simulink model "EGH446"  (R2020a)
settings: Solver=ode45  StartTime=0.0  StopTime=inf  RelTol=1e-5  EnableMultiTasking=on
PreLoadFcn:
  | ModelStartup
InitFcn:
  | load('sim_parameters')
  | load('complexMap.mat')
StartFcn:
  | drawPath
StopFcn:
  | drawPath
values from neighbouring files (symbols this model uses):
  dt = distanceTransform(x,[46,20])    [MapTest.m]
  obstacles = [4 8 8 8 2 14 22 16 23 24 12 21 ... (36 elements, 12x3)]    [obstacles.mat]
  path = [nodeRow(currentNode) nodeCol(currentNode); path]    [Astar.m]    (also in ModelStartup.m = [path(1:i-2,:); path(i:end,:)]; PathPlanning.m = [path; current])
  wpList = getWaypoints(NWaypoints,inflatedMap, obstacles, xmax,ymax)    [ModelStartup.m]
undefined symbols (not defined in the file or in its folder): DiscIntNeverNeededParam, Ke, mot_B, mot_COM, pp_cont, Ts, veh
libraries: mobileRoboticsLib x3, simulink_extras x3, simulink x3
PauseFcn:
  | drawPath
settings Model: SimulationMode=accelerator  Creator=sriramn  LastModifiedBy=CodyS
settings SolverCC: ZeroCrossAlgorithm=Adaptive
settings DataIOCC: LimitDataPoints=on  SaveFormat=Array  ReturnWorkspaceOutputs=off
settings OptimizationCC: LifeSpan=inf
settings DebuggingCC: SolverPrmCheckMsg=warning  AllowSymbolicDim=off  SFUnexpectedBacktrackingDiag=warning  SFNoUnconditionalDefaultTransitionDiag=warning  SFExecutionAtInitializationDiag=none  ArithmeticOperatorsInVariantConditions=warning
settings HardwareCC: ProdBitPerPointer=32  ProdBitPerSizeT=32  ProdBitPerPtrDiffT=32  ProdLargestAtomicFloat=None  ProdIntDivRoundTo=Undefined  ProdEndianess=Unspecified  ProdWordSize=32  ProdHWDeviceType=32-bit Generic
settings ModelReferenceCC: ModelReferenceMinAlgLoopOccurrences=on  PropagateSignalLabelsOutOfModel=off
settings SFSimCC: SimUseLocalCustomCode=off  CustomCodeUndefinedFunction=UseInterfaceOnly
settings RTWCC: RTWUseLocalCustomCode=off
settings CodeAppCC: StateflowObjectComments=on
settings GRTTargetCC: TargetLangStandard=C89/C90 (ANSI)
settings ConfigComp: CovMetricSettings=dw  CovHtmlReporting=on  CovSaveCumulativeToWorkspaceVar=on  CovSaveSingleToWorkspaceVar=on  CovExternalEMLEnable=off  CovSFcnEnable=off
settings SimscapeCC: SimscapeNormalizeSystem=off
settings ConfigurationSet: Description=SimMechanics 2G
settings ExplorerConfigSet: InternalSimMechanicsExplorerSettings="<ExplorerConfiguration><canonicalview>planar_xy</canonicalview><AnimationSetting><BasePlaybackSpeed>1.0</BasePlaybackSpeed><PlaybackSpeedFactor>1.0</PlaybackSpeedFactor></AnimationSetting><TilePanel><TileInfo><Tiles Columns=\"1\" Count=\"1\" Rows=\"1\"><Column Left=\"2\" Weight=\"1\"/><Column Left=\"1628\"/><Row Top=\"2\" Weight=\"1\"/><Row Top=\"1072\"/><Tile Height=\"1\" Width=\"1\" X=\"0\" Y=\"0\"/></Tiles></TileInfo><SceneInfo><SceneViewer><BGColor><R>0.60000002384185791</R><G>0.60000002384185791</G><B>0.60000002384185791</B></BGColor><Camera><Position><X>0.22951840878551699</X><Y>0.32651610611526627</Y><Z>-0.27215421354393321</Z></Position><Center><X>-0.15775714411666431</X><Y>-0.15462825985839526</Y><Z>0.065702552916005602</Z></Center><Up><X>-0.56030137557930915</X><Y>0.72817587161684794</Y><Z>0.39474329445726858</Z></Up><Left>-0.21481383955700509</Left><Right>0.21481383955700509</Right><Bottom>-0.27569784609469139</Bottom><Top>0.27569784609469139</Top></Camera></SceneViewer></SceneInfo></TilePanel></ExplorerConfiguration>"

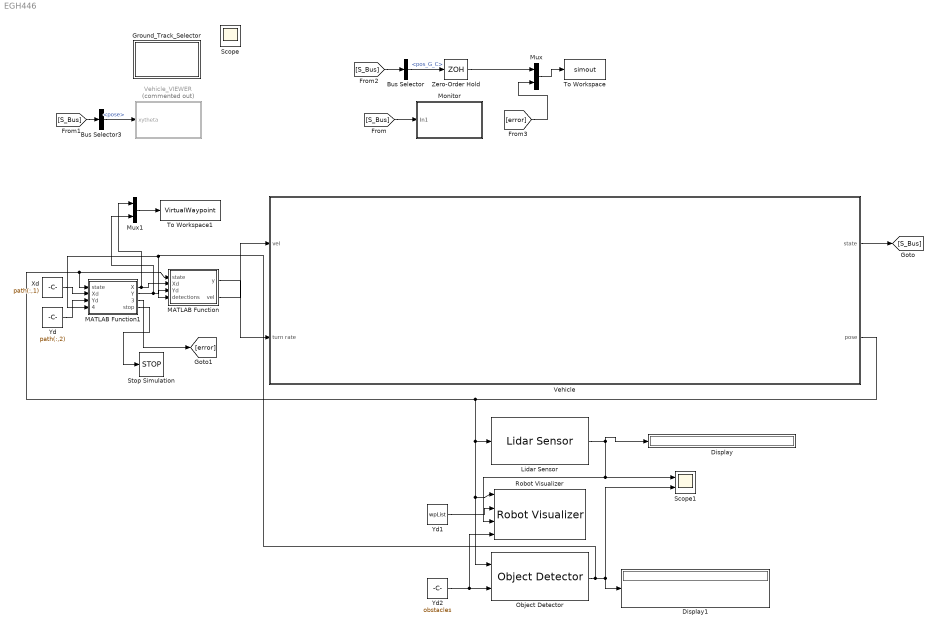
== system EGH446 ==
  Bus Selector : BusSelector  OutputSignals=BUS_G_frame.pos_G_C
  Bus Selector3 : BusSelector  OutputSignals=pose
  Display : Display
  Display1 : Display
  Ground_Track_Selector : Subsystem  mask{the_XL_filename=ground_robot_waypoints.xlsx, the_racetrack_str=SMALL_S_HOME, the_look_ahead_dist=0.260, the_des_lin_vel=0.1, the_max_ang_vel_deg_sec=60}
      mask prompts: the_XL_filename "EXCEL file (eg: bh.xlsx)"; the_racetrack_str "Racetrack type"; the_look_ahead_dist "Look ahead distance (m)"; the_des_lin_vel "Desired Linear Velocity (m/sec)"; the_max_ang_vel_deg_sec "Max Angular Velocity (deg/sec)"
      mask init:
      | %fprintf('\n ... <%s> and <%s>',the_XL_filename, the_racetrack_str);
      | 
      | A_MASK_OBJ  = Simulink.Mask.get(gcb);
      | A_IMAGE_OBJ = A_MASK_OBJ.getDialogControl('the_track_pic_param');
      | A_IMAGE_OBJ.FilePath = [the_racetrack_str,'.png'];
      | 
      | %--------------------------------------------------------------
      | THE_FILE  = the_XL_filename; 
      | THE_SHEET = the_racetrack_str;
      | my_path_data_T = readtable(THE_FILE, 'Sheet', THE_SHEET);
      | 
      | assignin('base', 'my_path_data_T', my_path_data_T );
      | evalin(  'base', 'pp_cont.Waypoints = [my_path_data_T.X,  my_path_data_T.Y ];' );
      | evalin('base', 'close all');
      | %--------------------------------------------------------------
      | evalin('base', ['pp_cont.LookaheadDistance=',num2str(the_look_ahead_dist),';']);
      | evalin('base', ['pp_cont.DesiredLinearVelocity=',num2str(the_des_lin_vel),';']);
      | evalin('base', ['pp_cont.MaxAngularVelocity=',num2str(the_max_ang_vel_deg_sec*pi/180),';']);
      | %pp_cont.LookaheadDistance     = 0.2;        % m 
      | %pp_cont.DesiredLinearVelocity = 0.1;        % m/s
      | %pp_cont.MaxAngularVelocity    = 60*pi/180;  %radians/second
      mask TypeOptions the_racetrack_str: SPANNER | RECT_TRI | MEDIUM_S_HOME | SMALL_S_HOME | SQUARE | CIRCLE_HOME | L_AND_R_TURNS | Assignment PartA | Tuning
      mask DialogControl DescGroupVar Prompt: m_RaceTrack_Selector
      mask DialogControl DescTextVar Prompt: Select the racetrack for your Differential Drive Robot (DDR).  And specify the parameters for your Pure Pursuit controller.
      mask DialogControl Container10 Prompt: RaceTrack
      mask DialogControl Container5 Prompt: PurePursuit
      mask DialogControl Control4 Prompt: If you want some DEFAULT values then click on the button below
      mask DialogControl the_set_def_PP_values Prompt: Set Default values
      mask DialogControl the_set_def_PP_values Callback:
      | set_param(gcb,'the_look_ahead_dist','0.2');
      | set_param(gcb,'the_des_lin_vel','0.1');
      | set_param(gcb,'the_max_ang_vel_deg_sec','60');
      | fprintf('\n *** applied DEFAULT values to PP params ***');
      mask DialogControl Control2 Prompt: As a general rule, the lookahead distance should be larger than the desired linear velocity for a smooth path. The robot might cut corners when the lookahead distance is large. In contrast, a small lookahead distance can result in an unstable path following behavior.
      mask Display: fprintf('%s',the_racetrack_str)
  Lidar Sensor : mobileRoboticsLib/Environments/Lidar Sensor  mapName=map  sensorOffset=[ 0, 0 ]  scanAngles=[ -pi/4, 0, pi/4 ]  maxRange=5
      settings: SourceProductName=Mobile Robotics Simulation Toolbox
  MATLAB Function : MATLAB Function  TreatAsAtomicUnit=on
  MATLAB Function1 : MATLAB Function  TreatAsAtomicUnit=on
  Monitor : Subsystem
  Mux : Mux  Inputs=2
  Mux1 : Mux  Inputs=2
  Object Detector : mobileRoboticsLib/Environments/Object Detector  sensorOffset=[ 0, 0 ]  sensorAngle=0  fieldOfView=pi/3  maxRange=5  maxDetections=3  sampleTime=0.1
      settings: SourceProductName=Mobile Robotics Simulation Toolbox
  Robot Visualizer : mobileRoboticsLib/Environments/Robot Visualizer  robotRadius=0  mapName=map  showTrajectory=on  hasWaypoints=on  hasLidar=on  sensorOffset=[ 0, 0 ]  scanAngles=[ -pi/4, 0, pi/4 ]  hasObjDetector=on  objDetectorOffset=[ 0, 0 ]  objDetectorAngle=0  objDetectorFOV=pi/4  objDetectorMaxRange=5  objectColors=[ 1, 0, 0; 0, 1, 0; 0, 0, 1 ]  objectMarkers=s
  Scope1 : Scope  NumInputPorts=2
  Stop Simulation : Stop
  To Workspace : ToWorkspace  VariableName=simout  SaveFormat=Structure With Time  SampleTime=-1
  To Workspace1 : ToWorkspace  VariableName=VirtualWaypoint  SampleTime=-1
  Vehicle : Subsystem
  Vehicle_VIEWER : Subsystem  Commented=on  mask{wp_mat=pp_cont.Waypoints, veh_ID_num=1, veh_init_xytheta=veh.states.init_pose, Ts=0.1}
      mask prompts: wp_mat "Waypoint matrix for arena [x_col, y_col] (m)"; veh_ID_num "Vehicle ID number"; veh_init_xytheta "Initial pose [x,y,theta]"; Ts "Sample time for updating animation (secs)"
      mask TypeOptions veh_ID_num: 1 | 2 | 3 | 4
      mask DialogControl Control2 Prompt: Animate simulation of Differential Drive Robot (DDR)
      mask Display: fprintf('veh_ID=%d',veh_ID_num);
  Xd : Constant  Value=path(:,1)
  Yd : Constant  Value=path(:,2)
  Yd1 : Constant  Value=wpList
  Yd2 : Constant  Value=obstacles
  Zero-Order Hold : ZeroOrderHold  SampleTime=0.01
  Scope : Scope
  wires:
  [S_Bus] -> Bus Selector3/1
  Bus Selector/1 -> Zero-Order Hold/1  "<pos_G_C>"
  Zero-Order Hold/1 -> Mux/1
  [S_Bus] -> Monitor/1(In1)
  Bus Selector3/1 -> Vehicle_VIEWER/1(xytheta)  "<pose>"
  [S_Bus] -> Bus Selector/1
  Vehicle/1(state) -> [S_Bus]
  MATLAB Function/1(y) -> Vehicle/2(turn rate)
  Vehicle/2(pose) -> Object Detector/1, Robot Visualizer/1, Lidar Sensor/1, MATLAB Function1/1(state), MATLAB Function/1(state)
  MATLAB Function/2(vel) -> Vehicle/1(vel)
  Xd/1 -> MATLAB Function1/2(Xd)
  Yd/1 -> MATLAB Function1/3(Yd)
  MATLAB Function1/1(X) -> Mux1/1, MATLAB Function/2(Xd)
  MATLAB Function1/2(Y) -> Mux1/2, MATLAB Function/3(Yd)
  MATLAB Function1/3(d_error) -> [error]
  MATLAB Function1/4(stop) -> Stop Simulation/1
  [error] -> Mux/2
  Mux/1 -> To Workspace/1
  Yd1/1 -> Robot Visualizer/2
  Yd2/1 -> Robot Visualizer/4, Object Detector/2
  Object Detector/1 -> MATLAB Function1/4(detections), MATLAB Function/4(detections), Scope1/2, Display1/1
  Lidar Sensor/1 -> Scope1/1, Robot Visualizer/3, Display/1
  Mux1/1 -> To Workspace1/1

== system EGH446/Ground_Track_Selector ==

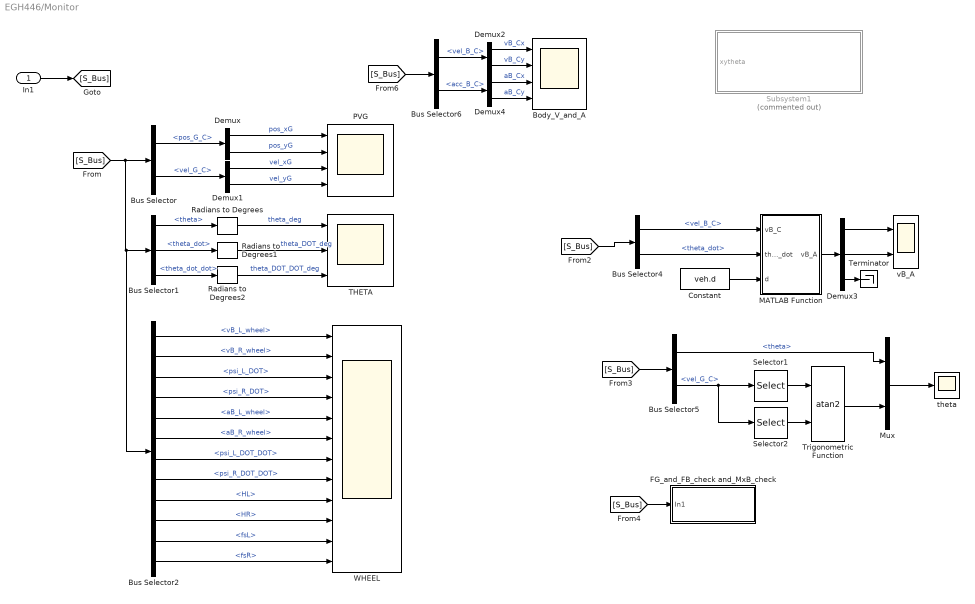
== system EGH446/Monitor ==
  In1 : Inport
  Body_V_and_A : Scope  NumInputPorts=4
  Bus Selector : BusSelector  OutputSignals=BUS_G_frame.pos_G_C,BUS_G_frame.vel_G_C
  Bus Selector1 : BusSelector  OutputSignals=theta,theta_dot,theta_dot_dot
  Bus Selector2 : BusSelector  OutputSignals=BUS_wheel.BUS_wheel_vel.vB_L_wheel,BUS_wheel.BUS_wheel_vel.vB_R_wheel,BUS_wheel.BUS_wheel_vel.psi_L_DOT,BUS_wheel.BUS_wheel_vel.psi_R_DOT,BUS_wheel.BUS_wheel_acc.aB_L_wheel,BUS_wheel.BUS_wheel_acc.aB_R_wheel,BUS_wheel.BUS_wheel_acc.psi_L_DOT_DOT,BUS_wheel.BUS_wheel_acc.psi_R_DOT_DOT,BUS_wheel.BUS_wheel_force.HL,BUS_wheel.BUS_wheel_force.HR,BUS_wheel.BUS_wheel_force.fsL,BUS_wheel.BUS_wheel_force.fsR
  Bus Selector4 : BusSelector  OutputSignals=BUS_B_frame.vel_B_C,theta_dot
  Bus Selector5 : BusSelector  OutputSignals=theta,BUS_G_frame.vel_G_C
  Bus Selector6 : BusSelector  OutputSignals=BUS_B_frame.vel_B_C,BUS_B_frame.acc_B_C
  Constant : Constant  Value=veh.d
  Demux{,1..2,4} (4 alike) : Demux  Outputs=2
  Demux3 : Demux  Outputs=3
  FG_and_FB_check and_MxB_check : Subsystem
  MATLAB Function : MATLAB Function  TreatAsAtomicUnit=on
  Mux : Mux  Inputs=2
  PVG : Scope  NumInputPorts=4
  Radians to Degrees : simulink_extras/Transformations/Radians to Degrees
  Radians to Degrees1 : simulink_extras/Transformations/Radians to Degrees
  Radians to Degrees2 : simulink_extras/Transformations/Radians to Degrees
  Selector1 : Selector  InputPortWidth=2  IndexOptions=Index vector (dialog)  Indices=[ 2]  OutputSizes=1
  Selector2 : Selector  InputPortWidth=2  IndexOptions=Index vector (dialog)  Indices=[ 1]  OutputSizes=1
  Subsystem1 : Subsystem  Commented=on  mask{wp_mat=[0, 1, 1, 0, 0, 1; 0,0,0.5,0.5,1,1]', veh_ID_num=2, veh_init_xytheta=[0,0,0], Ts=0.1}
      mask prompts: wp_mat "Waypoint matrix for arena [x_col, y_col] (m)"; veh_ID_num "Vehicle ID number"; veh_init_xytheta "Initial pose [x,y,theta]"; Ts "Sample time for updating animation (secs)"
      mask TypeOptions veh_ID_num: 1 | 2 | 3 | 4
      mask DialogControl Control2 Prompt: Animate simulation of Differential Drive Robot (DDR)
      mask Display: fprintf('veh_ID=%d',veh_ID_num);
  THETA : Scope  NumInputPorts=3
  Terminator : Terminator
  Trigonometric Function : Trigonometry  Operator=atan2
  WHEEL : Scope  NumInputPorts=12
  theta : Scope
  vB_A : Scope  NumInputPorts=2
  wires:
  In1/1 -> [S_Bus]
  [S_Bus] -> Bus Selector2/1, Bus Selector1/1, Bus Selector/1
  Bus Selector/1 -> Demux/1  "<pos_G_C>"
  Demux/1 -> PVG/1  "pos_xG"
  Demux/2 -> PVG/2  "pos_yG"
  Bus Selector/2 -> Demux1/1  "<vel_G_C>"
  Demux1/1 -> PVG/3  "vel_xG"
  Demux1/2 -> PVG/4  "vel_yG"
  Bus Selector1/1 -> Radians to Degrees/1  "<theta>"
  Radians to Degrees2/1 -> THETA/3  "theta_DOT_DOT_deg"
  Radians to Degrees1/1 -> THETA/2  "theta_DOT_deg"
  Radians to Degrees/1 -> THETA/1  "theta_deg"
  Bus Selector1/2 -> Radians to Degrees1/1  "<theta_dot>"
  Bus Selector1/3 -> Radians to Degrees2/1  "<theta_dot_dot>"
  Bus Selector2/5 -> WHEEL/5  "<aB_L_wheel>"
  Bus Selector2/9 -> WHEEL/9  "<HL>"
  Bus Selector2/7 -> WHEEL/7  "<psi_L_DOT_DOT>"
  Bus Selector2/2 -> WHEEL/2  "<vB_R_wheel>"
  Bus Selector2/4 -> WHEEL/4  "<psi_R_DOT>"
  Bus Selector2/6 -> WHEEL/6  "<aB_R_wheel>"
  Bus Selector2/8 -> WHEEL/8  "<psi_R_DOT_DOT>"
  Bus Selector2/3 -> WHEEL/3  "<psi_L_DOT>"
  Bus Selector2/1 -> WHEEL/1  "<vB_L_wheel>"
  Bus Selector2/10 -> WHEEL/10  "<HR>"
  Bus Selector2/11 -> WHEEL/11  "<fsL>"
  Bus Selector2/12 -> WHEEL/12  "<fsR>"
  [S_Bus] -> Bus Selector4/1
  Bus Selector4/1 -> MATLAB Function/1(vB_C)  "<vel_B_C>"
  [S_Bus] -> Bus Selector5/1
  Bus Selector5/2 -> Selector1/1, Selector2/1  "<vel_G_C>"
  Selector2/1 -> Trigonometric Function/2
  Selector1/1 -> Trigonometric Function/1
  Trigonometric Function/1 -> Mux/2
  Bus Selector5/1 -> Mux/1  "<theta>"
  Mux/1 -> theta/1
  Bus Selector4/2 -> MATLAB Function/2(theta_dot)  "<theta_dot>"
  Constant/1 -> MATLAB Function/3(d)
  MATLAB Function/1(vB_A) -> Demux3/1
  Demux3/3 -> Terminator/1
  Demux3/1 -> vB_A/1
  Demux3/2 -> vB_A/2
  [S_Bus] -> Bus Selector6/1
  Demux4/1 -> Body_V_and_A/3  "aB_Cx"
  Demux4/2 -> Body_V_and_A/4  "aB_Cy"
  Bus Selector6/1 -> Demux2/1  "<vel_B_C>"
  Bus Selector6/2 -> Demux4/1  "<acc_B_C>"
  Demux2/2 -> Body_V_and_A/2  "vB_Cy"
  Demux2/1 -> Body_V_and_A/1  "vB_Cx"
  [S_Bus] -> FG_and_FB_check and_MxB_check/1(In1)

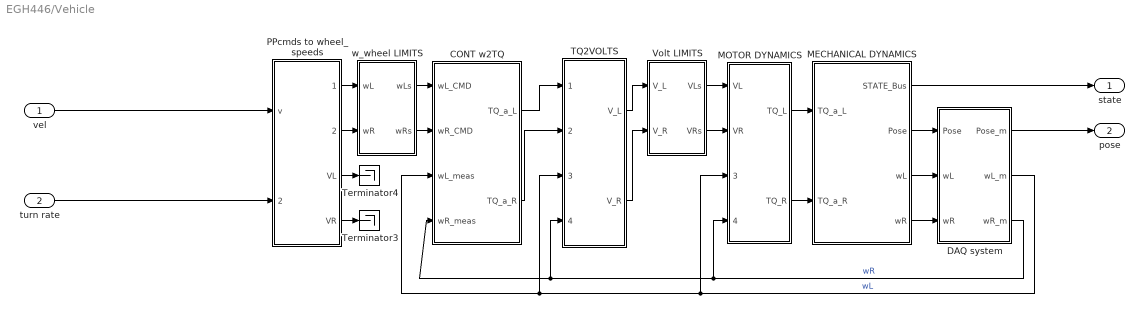
== system EGH446/Vehicle ==
  vel : Inport
  turn rate : Inport  Port=2
  CONT w2TQ : Subsystem
  DAQ system : Subsystem
  MECHANICAL DYNAMICS : Subsystem
      mask Display: image(imread('bh_pics_veh_01.JPG'));
  MOTOR DYNAMICS : Subsystem
  PPcmds to wheel_speeds : Subsystem  mask(PP_cmds_to_Wheel_vels){r=veh.wheel.r, L=veh.L_half_axle}
      mask prompts: r "Radius (r) of driving wheels (m)"; L "Axle HALF length (L) separating wheels  (m)"
      mask help: Convert Pure Pursuit commands into WHEEL velocities.
      mask DialogControl Container10 Prompt: GEOMETRY
  TQ2VOLTS : Subsystem
  Terminator3 : Terminator
  Terminator4 : Terminator
  Volt LIMITS : Subsystem
      mask Display: image(imread('bh_sat.JPG'), [0.25 0.25 0.5 0.5])
  w_wheel LIMITS : Subsystem
      mask Display: image(imread('bh_sat.JPG'), [0.25 0.25 0.5 0.5])
  state : Outport  VectorParamsAs1DForOutWhenUnconnected=off
  pose : Outport  Port=2  VectorParamsAs1DForOutWhenUnconnected=off
  wires:
  turn rate/1 -> PPcmds to wheel_speeds/2(theta_DOT)
  vel/1 -> PPcmds to wheel_speeds/1(v)
  PPcmds to wheel_speeds/4(VR) -> Terminator3/1
  CONT w2TQ/1(TQ_a_L) -> TQ2VOLTS/1(TL_cmd)
  TQ2VOLTS/2(V_R) -> Volt LIMITS/2(V_R)
  DAQ system/1(Pose_m) -> pose/1
  MOTOR DYNAMICS/2(TQ_R) -> MECHANICAL DYNAMICS/2(TQ_a_R)
  Volt LIMITS/1(VLs) -> MOTOR DYNAMICS/1(VL)
  PPcmds to wheel_speeds/3(VL) -> Terminator4/1
  PPcmds to wheel_speeds/1(wL_wheel) -> w_wheel LIMITS/1(wL)
  TQ2VOLTS/1(V_L) -> Volt LIMITS/1(V_L)
  MECHANICAL DYNAMICS/1(STATE_Bus) -> state/1
  Volt LIMITS/2(VRs) -> MOTOR DYNAMICS/2(VR)
  w_wheel LIMITS/2(wRs) -> CONT w2TQ/2(wR_CMD)
  w_wheel LIMITS/1(wLs) -> CONT w2TQ/1(wL_CMD)
  DAQ system/3(wR_m) -> CONT w2TQ/4(wR_meas), TQ2VOLTS/4(wR_meas), MOTOR DYNAMICS/4(wR_meas)  "wR"
  CONT w2TQ/2(TQ_a_R) -> TQ2VOLTS/2(TR_cmd)
  MECHANICAL DYNAMICS/3(wL) -> DAQ system/2(wL)
  MOTOR DYNAMICS/1(TQ_L) -> MECHANICAL DYNAMICS/1(TQ_a_L)
  MECHANICAL DYNAMICS/2(Pose) -> DAQ system/1(Pose)
  DAQ system/2(wL_m) -> CONT w2TQ/3(wL_meas), TQ2VOLTS/3(wL_meas), MOTOR DYNAMICS/3(wL_meas)  "wL"
  PPcmds to wheel_speeds/2(wR_wheel) -> w_wheel LIMITS/2(wR)
  MECHANICAL DYNAMICS/4(wR) -> DAQ system/3(wR)

== system EGH446/Vehicle_VIEWER ==
  xytheta : Inport
  Level-2 MATLAB S-Function : M-S-Function  FunctionName=bh_ddr_animate_sfun  Parameters=Ts, wp_mat, veh_ID_num, veh_init_xytheta
  Signal Specification : SignalSpecification  Dimensions=3
  wires:
  xytheta/1 -> Signal Specification/1
  Signal Specification/1 -> Level-2 MATLAB S-Function/1

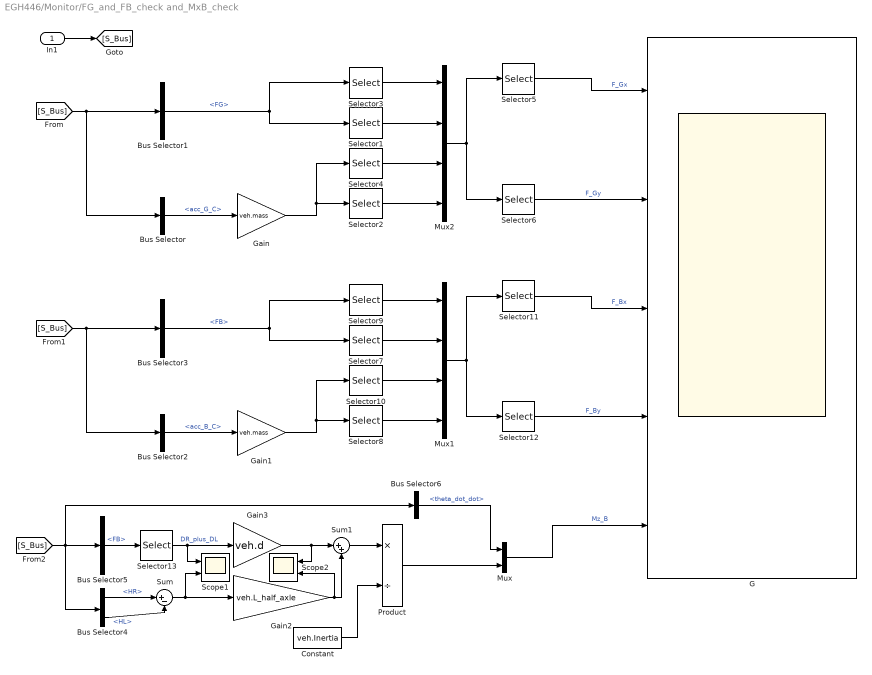
== system EGH446/Monitor/FG_and_FB_check and_MxB_check ==
  In1 : Inport
  Bus Selector : BusSelector  OutputSignals=BUS_G_frame.acc_G_C
  Bus Selector1 : BusSelector  OutputSignals=BUS_veh_F.BUS_veh_FG.FG
  Bus Selector2 : BusSelector  OutputSignals=BUS_B_frame.acc_B_C
  Bus Selector3 : BusSelector  OutputSignals=BUS_veh_F.BUS_veh_Fb.FB
  Bus Selector4 : BusSelector  OutputSignals=BUS_wheel.BUS_wheel_force.HR,BUS_wheel.BUS_wheel_force.HL
  Bus Selector5 : BusSelector  OutputSignals=BUS_veh_F.BUS_veh_Fb.FB
  Bus Selector6 : BusSelector  OutputSignals=theta_dot_dot
  Constant : Constant  Value=veh.Inertia
  G : Scope  NumInputPorts=5
  Gain : Gain  Gain=veh.mass
  Gain1 : Gain  Gain=veh.mass
  Gain2 : Gain  Gain=veh.L_half_axle
  Gain3 : Gain  Gain=veh.d
  Mux : Mux  Inputs=2
  Mux1 : Mux
  Mux2 : Mux
  Product : Product  Inputs=*/
  Scope1 : Scope  NumInputPorts=2
  Scope2 : Scope  NumInputPorts=2
  Selector{1..2,7..8,13} (5 alike) : Selector  InputPortWidth=2  IndexOptions=Index vector (dialog)  Indices=2  OutputSizes=1
  Selector{3..4,9..10} (4 alike) : Selector  InputPortWidth=2  IndexOptions=Index vector (dialog)  Indices=1  OutputSizes=1
  Selector11 : Selector  InputPortWidth=4  IndexOptions=Index vector (dialog)  Indices=[1 3]  OutputSizes=1
  Selector12 : Selector  InputPortWidth=4  IndexOptions=Index vector (dialog)  Indices=[2 4]  OutputSizes=1
  Selector5 : Selector  InputPortWidth=4  IndexOptions=Index vector (dialog)  Indices=[1 3]  OutputSizes=1
  Selector6 : Selector  InputPortWidth=4  IndexOptions=Index vector (dialog)  Indices=[2 4]  OutputSizes=1
  Sum : Sum  Inputs=|+-
  Sum1 : Sum  Inputs=|++
  wires:
  In1/1 -> [S_Bus]
  [S_Bus] -> Bus Selector/1, Bus Selector1/1
  Bus Selector/1 -> Gain/1  "<acc_G_C>"
  Gain/1 -> Selector4/1, Selector2/1
  Selector3/1 -> Mux2/1
  Selector1/1 -> Mux2/2
  Selector4/1 -> Mux2/3
  Selector2/1 -> Mux2/4
  Mux2/1 -> Selector5/1, Selector6/1
  Selector6/1 -> G/2  "F_Gy"
  Selector5/1 -> G/1  "F_Gx"
  Bus Selector1/1 -> Selector3/1, Selector1/1  "<FG>"
  [S_Bus] -> Bus Selector2/1, Bus Selector3/1
  Bus Selector2/1 -> Gain1/1  "<acc_B_C>"
  Gain1/1 -> Selector10/1, Selector8/1
  Selector9/1 -> Mux1/1
  Selector7/1 -> Mux1/2
  Selector10/1 -> Mux1/3
  Selector8/1 -> Mux1/4
  Mux1/1 -> Selector11/1, Selector12/1
  Selector12/1 -> G/4  "F_By"
  Selector11/1 -> G/3  "F_Bx"
  Bus Selector3/1 -> Selector9/1, Selector7/1  "<FB>"
  [S_Bus] -> Bus Selector6/1, Bus Selector4/1, Bus Selector5/1
  Bus Selector5/1 -> Selector13/1  "<FB>"
  Selector13/1 -> Scope1/1, Gain3/1  "DR_plus_DL"
  Sum/1 -> Scope1/2, Gain2/1
  Gain3/1 -> Scope2/1, Sum1/1
  Gain2/1 -> Scope2/2, Sum1/2
  Mux/1 -> G/5  "Mz_B"
  Product/1 -> Mux/2
  Constant/1 -> Product/2
  Sum1/1 -> Product/1
  Bus Selector4/1 -> Sum/1  "<HR>"
  Bus Selector4/2 -> Sum/2  "<HL>"
  Bus Selector6/1 -> Mux/1  "<theta_dot_dot>"

== system EGH446/Monitor/Subsystem1 ==
  xytheta : Inport
  Level-2 MATLAB S-Function : M-S-Function  FunctionName=bh_ddr_animate_sfun  Parameters=Ts, wp_mat, veh_ID_num, veh_init_xytheta
  Signal Specification : SignalSpecification  Dimensions=3
  wires:
  xytheta/1 -> Signal Specification/1
  Signal Specification/1 -> Level-2 MATLAB S-Function/1

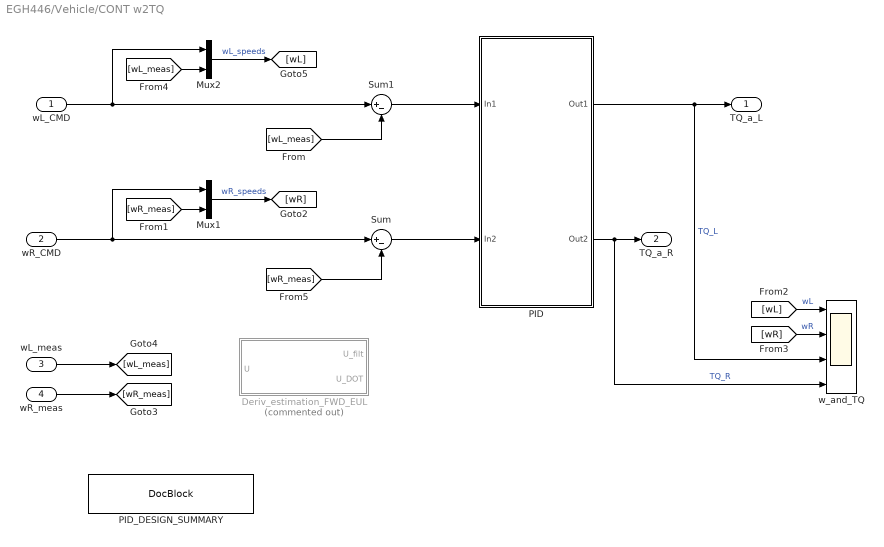
== system EGH446/Vehicle/CONT w2TQ ==
  wL_CMD : Inport
  wR_CMD : Inport  Port=2
  wL_meas : Inport  Port=3
  wR_meas : Inport  Port=4
  Deriv_estimation_FWD_EUL : Subsystem  Commented=on  mask(Derivative Estimation){wn=2*pi*15, p=1, dt=dt}
      mask prompts: wn "Natural frequency, wn (rad/sec)"; p "Damping ratio, p"; dt "Sample time, dt (secs)"
      mask help:
      | A simple derivative estimator using a 2nd order representation between input and output.
      |
      | The integrators use a discrete FORWARd Euler rule, and a sample time needs to be specified.
      mask init:
      | str1 = sprintf('wn = %.2f', wn);
      | str2 = sprintf('p  = %.2f', p);
      | str3 = sprintf('dt = %.2f', dt);
      | str = char(str1,str2,str3);
      mask Display: disp(str)
  Mux1 : Mux  Inputs=2
  Mux2 : Mux  Inputs=2
  PID : Subsystem  mask{kp=0.01, ki=0, kd=0, dt=dt}
      mask prompts: dt "dt (secs)"
  PID_DESIGN_SUMMARY : simulink/Model-Wide Utilities/DocBlock  DocumentType=Text
      content=|
      | DESIGNS:
      |
      | dt=0.01
      |
      | 1.)  p=1e-2,  i=0,     d=0
      | 2.)  p=0.029, i=0.034, d=0
      | ++++++++++++++++++++++++++++++++++++++++++++++++++++++
  Sum : Sum  Inputs=|+-
  Sum1 : Sum  Inputs=|+-
  w_and_TQ : Scope  NumInputPorts=4
  TQ_a_L : Outport  VectorParamsAs1DForOutWhenUnconnected=off
  TQ_a_R : Outport  Port=2  VectorParamsAs1DForOutWhenUnconnected=off
  wires:
  Sum1/1 -> PID/1(In1)
  Sum/1 -> PID/2(In2)
  [wR_meas] -> Mux1/2
  PID/1(Out1) -> w_and_TQ/3, TQ_a_L/1  "TQ_L"
  Mux1/1 -> [wR]  "wR_speeds"
  [wL] -> w_and_TQ/1  "wL"
  [wR] -> w_and_TQ/2  "wR"
  wR_CMD/1 -> Mux1/1, Sum/1
  wR_meas/1 -> [wR_meas]
  wL_meas/1 -> [wL_meas]
  [wL_meas] -> Mux2/2
  Mux2/1 -> [wL]  "wL_speeds"
  wL_CMD/1 -> Sum1/1, Mux2/1
  [wL_meas] -> Sum1/2
  [wR_meas] -> Sum/2
  PID/2(Out2) -> TQ_a_R/1, w_and_TQ/4  "TQ_R"

== system EGH446/Vehicle/DAQ system ==
  Pose : Inport
  wL : Inport  Port=2
  wR : Inport  Port=3
  LPF : Subsystem  mask{fc=(2/3)*(1/Ts)*0.5}
      mask prompts: fc "LPF cutoff Frequency (Hz)"
      mask Display: fprintf('LPF\n fc = %.0f (Hz)', fc);
  Zero-Order Hold : ZeroOrderHold  SampleTime=Ts
      settings: AttributesFormatString=Ts=%<SampleTime>
  Zero-Order Hold1 : ZeroOrderHold  SampleTime=Ts
      settings: AttributesFormatString=Ts=%<SampleTime>
  Zero-Order Hold2 : ZeroOrderHold  SampleTime=Ts
      settings: AttributesFormatString=Ts=%<SampleTime>
  Pose_m : Outport  VectorParamsAs1DForOutWhenUnconnected=off
  wL_m : Outport  Port=2  VectorParamsAs1DForOutWhenUnconnected=off
  wR_m : Outport  Port=3  VectorParamsAs1DForOutWhenUnconnected=off
  wires:
  Zero-Order Hold/1 -> Pose_m/1
  Zero-Order Hold1/1 -> wL_m/1
  Zero-Order Hold2/1 -> wR_m/1
  Pose/1 -> LPF/1(Pose)
  wL/1 -> LPF/2(wL)
  wR/1 -> LPF/3(wR)
  LPF/3(wR_m) -> Zero-Order Hold2/1
  LPF/2(wL_m) -> Zero-Order Hold1/1
  LPF/1(Pose_m) -> Zero-Order Hold/1

== system EGH446/Vehicle/MECHANICAL DYNAMICS ==
  TQ_a_L : Inport
  TQ_a_R : Inport  Port=2
  DDR_SYS : ModelReference  ModelNameDialog=bh_DDR_component_model.slx  SimulationMode=Normal  ModelReferenceVersion=1.697
  STATE_Bus : Outport  VectorParamsAs1DForOutWhenUnconnected=off
  Pose : Outport  Port=2  VectorParamsAs1DForOutWhenUnconnected=off
  wL : Outport  Port=3  VectorParamsAs1DForOutWhenUnconnected=off
  wR : Outport  Port=4  VectorParamsAs1DForOutWhenUnconnected=off
  wires:
  DDR_SYS/4 -> wR/1
  DDR_SYS/3 -> wL/1
  DDR_SYS/2 -> Pose/1
  DDR_SYS/1 -> STATE_Bus/1
  TQ_a_R/1 -> DDR_SYS/2
  TQ_a_L/1 -> DDR_SYS/1

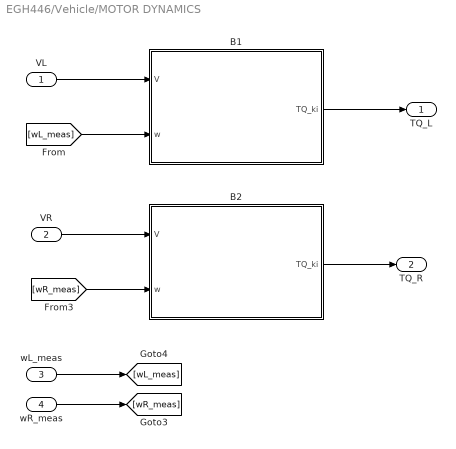
== system EGH446/Vehicle/MOTOR DYNAMICS ==
  VL : Inport
  VR : Inport  Port=2
  wL_meas : Inport  Port=3
  wR_meas : Inport  Port=4
  B1 : Subsystem  mask(DC motor (w_IN and TQ_out)){R=mot_B.R, K=mot_B.K, Kb=Ke}
      mask prompts: R "Armature resistance (ohms)"; K "Torque constant (N.m/A)"; Kb "Back Emf constant (V.sec/rad)"
      mask help: A DC motor model that outputs TORQUE for a given speed input
      mask DialogControl Control2 Prompt: NOTE:  with SI units, the Toque constant (Ka) and Back EMF constant(Kb) are the same.
      mask DialogControl Container9 Prompt: Electrical
      mask Display: fprintf('DC motor\n(w_IN \n and \n TQ_out)');
  B2 : Subsystem  mask(DC motor (w_IN and TQ_out)){R=mot_B.R, K=mot_B.K, Kb=Ke}
      mask prompts: R "Armature resistance (ohms)"; K "Torque constant (N.m/A)"; Kb "Back Emf constant (V.sec/rad)"
      mask help: A DC motor model that outputs TORQUE for a given speed input
      mask DialogControl Control2 Prompt: NOTE:  with SI units, the Toque constant (Ka) and Back EMF constant(Kb) are the same.
      mask DialogControl Container9 Prompt: Electrical
      mask Display: fprintf('DC motor\n(w_IN \n and \n TQ_out)');
  TQ_L : Outport  VectorParamsAs1DForOutWhenUnconnected=off
  TQ_R : Outport  Port=2  VectorParamsAs1DForOutWhenUnconnected=off
  wires:
  wR_meas/1 -> [wR_meas]
  wL_meas/1 -> [wL_meas]
  B1/1(TQ_ki) -> TQ_L/1
  B2/1(TQ_ki) -> TQ_R/1
  [wL_meas] -> B1/2(w)
  VL/1 -> B1/1(V)
  [wR_meas] -> B2/2(w)
  VR/1 -> B2/1(V)

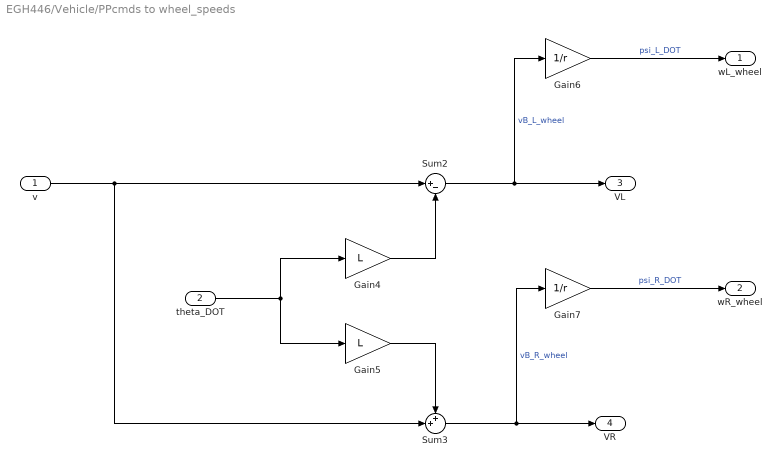
== system EGH446/Vehicle/PPcmds to wheel_speeds ==
  v : Inport
  theta_DOT : Inport  Port=2
  Gain4 : Gain  Gain=L
  Gain5 : Gain  Gain=L
  Gain6 : Gain  Gain=1/r
  Gain7 : Gain  Gain=1/r
  Sum2 : Sum  Inputs=|+-
  Sum3 : Sum  Inputs=++|
  wL_wheel : Outport  VectorParamsAs1DForOutWhenUnconnected=off
  wR_wheel : Outport  Port=2  VectorParamsAs1DForOutWhenUnconnected=off
  VL : Outport  Port=3  VectorParamsAs1DForOutWhenUnconnected=off
  VR : Outport  Port=4  VectorParamsAs1DForOutWhenUnconnected=off
  wires:
  v/1 -> Sum3/2, Sum2/1
  theta_DOT/1 -> Gain4/1, Gain5/1
  Gain4/1 -> Sum2/2
  Sum2/1 -> VL/1, Gain6/1  "vB_L_wheel"
  Gain5/1 -> Sum3/1
  Sum3/1 -> VR/1, Gain7/1  "vB_R_wheel"
  Gain6/1 -> wL_wheel/1  "psi_L_DOT"
  Gain7/1 -> wR_wheel/1  "psi_R_DOT"

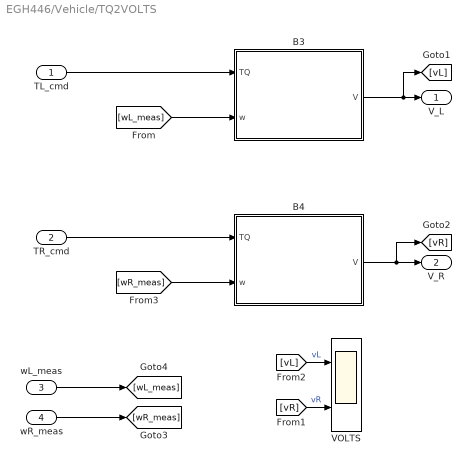
== system EGH446/Vehicle/TQ2VOLTS ==
  TL_cmd : Inport
  TR_cmd : Inport  Port=2
  wL_meas : Inport  Port=3
  wR_meas : Inport  Port=4
  B3 : Subsystem  mask(DC motor (w_IN and TQ_out)){R=mot_B.R, K=mot_B.K, Kb=Ke}
      mask prompts: R "Armature resistance (ohms)"; K "Torque constant (N.m/A)"; Kb "Back Emf constant (V.sec/rad)"
      mask help: A DC motor model that outputs TORQUE for a given speed input
      mask DialogControl Control2 Prompt: NOTE:  with SI units, the Toque constant (Ka) and Back EMF constant(Kb) are the same.
      mask DialogControl Container9 Prompt: Electrical
      mask Display: fprintf('DC motor\n(TQ_IN \n and \n V_out)');
  B4 : Subsystem  mask(DC motor (w_IN and TQ_out)){R=mot_B.R, K=mot_B.K, Kb=Ke}
      mask prompts: R "Armature resistance (ohms)"; K "Torque constant (N.m/A)"; Kb "Back Emf constant (V.sec/rad)"
      mask help: A DC motor model that outputs TORQUE for a given speed input
      mask DialogControl Control2 Prompt: NOTE:  with SI units, the Toque constant (Ka) and Back EMF constant(Kb) are the same.
      mask DialogControl Container9 Prompt: Electrical
      mask Display: fprintf('DC motor\n(TQ_IN \n and \n V_out)');
  VOLTS : Scope  NumInputPorts=2
  V_L : Outport  VectorParamsAs1DForOutWhenUnconnected=off
  V_R : Outport  Port=2  VectorParamsAs1DForOutWhenUnconnected=off
  wires:
  wR_meas/1 -> [wR_meas]
  wL_meas/1 -> [wL_meas]
  TL_cmd/1 -> B3/1(TQ)
  [wL_meas] -> B3/2(w)
  B3/1(V) -> [vL], V_L/1
  TR_cmd/1 -> B4/1(TQ)
  [wR_meas] -> B4/2(w)
  B4/1(V) -> [vR], V_R/1
  [vL] -> VOLTS/1  "vL"
  [vR] -> VOLTS/2  "vR"

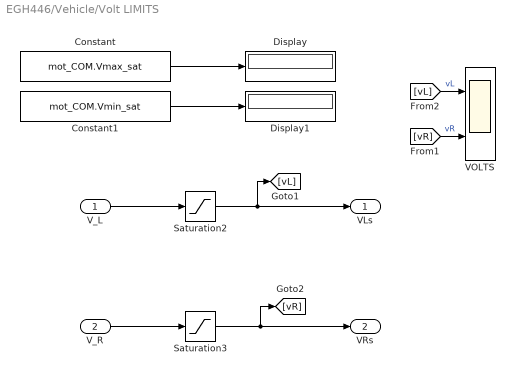
== system EGH446/Vehicle/Volt LIMITS ==
  V_L : Inport
  V_R : Inport  Port=2
  Constant : Constant  Value=mot_COM.Vmax_sat
  Constant1 : Constant  Value=mot_COM.Vmin_sat
  Display : Display
  Display1 : Display
  Saturation2 : Saturate  UpperLimit=mot_COM.Vmax_sat  LowerLimit=mot_COM.Vmin_sat
      settings: AttributesFormatString=|
      | %<UpperLimit>
      | %<LowerLimit>
  Saturation3 : Saturate  UpperLimit=mot_COM.Vmax_sat  LowerLimit=mot_COM.Vmin_sat
      settings: AttributesFormatString=|
      | %<UpperLimit>
      | %<LowerLimit>
  VOLTS : Scope  NumInputPorts=2
  VLs : Outport  VectorParamsAs1DForOutWhenUnconnected=off
  VRs : Outport  Port=2  VectorParamsAs1DForOutWhenUnconnected=off
  wires:
  V_L/1 -> Saturation2/1
  Saturation2/1 -> [vL], VLs/1
  Saturation3/1 -> [vR], VRs/1
  V_R/1 -> Saturation3/1
  Constant1/1 -> Display1/1
  Constant/1 -> Display/1
  [vL] -> VOLTS/1  "vL"
  [vR] -> VOLTS/2  "vR"

== system EGH446/Vehicle/w_wheel LIMITS ==
  wL : Inport
  wR : Inport  Port=2
  Constant : Constant  Value=mot_COM.w_max
  Constant1 : Constant  Value=-1*mot_COM.w_max
  Dashboard Scope : DashboardScope
  Dashboard Scope1 : DashboardScope
  Display : Display
  Display1 : Display
  Saturation : Saturate  UpperLimit=mot_COM.w_max  LowerLimit=-1*mot_COM.w_max
      settings: AttributesFormatString=|
      | wmax = %<UpperLimit>
      | wmin = %<LowerLimit>
  Saturation1 : Saturate  UpperLimit=mot_COM.w_max  LowerLimit=-1*mot_COM.w_max
      settings: AttributesFormatString=|
      | wmax = %<UpperLimit>
      | wmin = %<LowerLimit>
  wLs : Outport  VectorParamsAs1DForOutWhenUnconnected=off
  wRs : Outport  Port=2  VectorParamsAs1DForOutWhenUnconnected=off
  wires:
  wL/1 -> Saturation/1
  wR/1 -> Saturation1/1
  Saturation1/1 -> wRs/1
  Saturation/1 -> wLs/1
  Constant/1 -> Display/1
  Constant1/1 -> Display1/1

== system EGH446/Vehicle/CONT w2TQ/Deriv_estimation_FWD_EUL ==
  note: Y = U *     wn^2/( s^2 + 2*p*wn*s + wn^2)
      | Y*( s^2 + 2*p*wn*s + wn^2) = U * wn^2
      |
      | y'' + y'*2*p*wn + y*wn^2 = U*wn^2
  U : Inport
  Discrete-Time Integrator : DiscreteIntegrator  SampleTime=dt  ICPrevOutput=DiscIntNeverNeededParam  ICPrevScaledInput=DiscIntNeverNeededParam
  Discrete-Time Integrator1 : DiscreteIntegrator  SampleTime=dt  ICPrevOutput=DiscIntNeverNeededParam  ICPrevScaledInput=DiscIntNeverNeededParam
  Gain : Gain  Gain=2*p*wn
  Gain1 : Gain  Gain=wn^2
  Gain2 : Gain  Gain=wn^2
  Sum : Sum  Inputs=|+--
  U_filt : Outport  VectorParamsAs1DForOutWhenUnconnected=off
  U_DOT : Outport  Port=2  VectorParamsAs1DForOutWhenUnconnected=off
  wires:
  Discrete-Time Integrator1/1 -> Discrete-Time Integrator/1, [Y_DOT], Gain/1  "y_dot"
  Sum/1 -> Discrete-Time Integrator1/1  "y_dot_dot"
  Discrete-Time Integrator/1 -> Gain1/1, U_filt/1  "y"
  U/1 -> Gain2/1
  Gain2/1 -> Sum/1
  Gain/1 -> Sum/3
  Gain1/1 -> Sum/2
  [Y_DOT] -> U_DOT/1

== system EGH446/Vehicle/CONT w2TQ/PID ==
  In1 : Inport
  In2 : Inport  Port=2
  PID_L : simulink/Continuous/PID Controller  Controller=PID  Form=Parallel  TimeDomain=Discrete-time  UseExternalTs=off  SampleTime=dt  IntegratorMethod=Forward Euler  FilterMethod=Forward Euler  ControllerParametersSource=internal  P=kp  I=ki  D=kd  UseFilter=on  N=100  TunerSelectOption=Transfer Function Based (PID Tuner App)  InitialConditionSource=internal  InitialConditionForIntegrator=0  InitialConditionForFilter=0  DifferentiatorICPrevScaledInput=0  ExternalReset=none  TrackingMode=off  Kt=1  LimitOutput=off  UpperSaturationLimit=inf  LowerSaturationLimit=-inf  LinearizeAsGain=on  AntiWindupMode=none  Kb=1  POutMin=[]  POutMax=[]  IOutMin=[]  IOutMax=[]  DOutMin=[]  DOutMax=[]  NOutMin=[]  NOutMax=[]  SumOutMin=[]  SumOutMax=[]  SaturationOutMin=[]  SaturationOutMax=[]  PParamMin=[]  PParamMax=[]  IParamMin=[]  IParamMax=[]  DParamMin=[]  DParamMax=[]  NParamMin=[]  NParamMax=[]  KbParamMin=[]  KbParamMax=[]  KtParamMin=[]  KtParamMax=[]  KbOutMin=[]  KbOutMax=[]  KtOutMin=[]  KtOutMax=[]  IntegratorOutMin=[]  IntegratorOutMax=[]  FilterOutMin=[]  FilterOutMax=[]  SumI1OutMin=[]  SumI1OutMax=[]  SumI2OutMin=[]  SumI2OutMax=[]  SumI3OutMin=[]  SumI3OutMax=[]  SumI4OutMin=[]  SumI4OutMax=[]  SumDOutMin=[]  SumDOutMax=[]  DifferentiatorOutMin=[]  DifferentiatorOutMax=[]  FilterDiffOutCoefMin=[]  FilterDiffOutCoefMax=[]  ReciprocalOutMin=[]  ReciprocalOutMax=[]  SumDenOutMin=[]  SumDenOutMax=[]  SumNumOutMin=[]  SumNumOutMax=[]  DivideOutMin=[]  DivideOutMax=[]  UdiffTsProdOutMin=[]  UdiffTsProdOutMax=[]  NTsProdOutMin=[]  NTsProdOutMax=[]  UintegralTsProdOutMin=[]  UintegralTsProdOutMax=[]  UngainTsProdOutMin=[]  UngainTsProdOutMax=[]  IntegratorContinuousStateAttributes=''  IntegratorStateMustResolveToSignalObject=off  IntegratorRTWStateStorageClass=Auto  FilterContinuousStateAttributes=''  FilterStateMustResolveToSignalObject=off  FilterRTWStateStorageClass=Auto  ParallelPVariant=InternalParameters  IdealPVariant=Disabled  IVariant=InternalParameters  DVariant=InternalParameters  IntegratorVariant=Discrete  SatVariant=Disabled  AWVariant=Passthrough  PCopyVariant=Disabled  TRVariant=Disabled  FdbkBlocksVariant=Forward  IdealPFdbkVariant=Disabled  SatFdbkVariant=Disabled  DerivativeFilterVariant=ForwardEulerFilter  NVariant=InternalParameters  NCopyVariant=Disabled  FilterICVariant=InternalICsFilter  IntegratorICVariant=InternalICs  ExternalResetVariant=Disabled  TRSumVariant=Passthrough  SumFdbkVariant=Disabled  SumVariant=Sum_PID  TsampFilterVariant=InternalTs  TsampNgainVariant=Passthrough  TsampIntegralVariant=Passthrough
  PID_R : simulink/Continuous/PID Controller  Controller=PID  Form=Parallel  TimeDomain=Discrete-time  UseExternalTs=off  SampleTime=dt  IntegratorMethod=Forward Euler  FilterMethod=Forward Euler  ControllerParametersSource=internal  P=kp  I=ki  D=kd  UseFilter=on  N=100  TunerSelectOption=Transfer Function Based (PID Tuner App)  InitialConditionSource=internal  InitialConditionForIntegrator=0  InitialConditionForFilter=0  DifferentiatorICPrevScaledInput=0  ExternalReset=none  TrackingMode=off  Kt=1  LimitOutput=off  UpperSaturationLimit=inf  LowerSaturationLimit=-inf  LinearizeAsGain=on  AntiWindupMode=none  Kb=1  POutMin=[]  POutMax=[]  IOutMin=[]  IOutMax=[]  DOutMin=[]  DOutMax=[]  NOutMin=[]  NOutMax=[]  SumOutMin=[]  SumOutMax=[]  SaturationOutMin=[]  SaturationOutMax=[]  PParamMin=[]  PParamMax=[]  IParamMin=[]  IParamMax=[]  DParamMin=[]  DParamMax=[]  NParamMin=[]  NParamMax=[]  KbParamMin=[]  KbParamMax=[]  KtParamMin=[]  KtParamMax=[]  KbOutMin=[]  KbOutMax=[]  KtOutMin=[]  KtOutMax=[]  IntegratorOutMin=[]  IntegratorOutMax=[]  FilterOutMin=[]  FilterOutMax=[]  SumI1OutMin=[]  SumI1OutMax=[]  SumI2OutMin=[]  SumI2OutMax=[]  SumI3OutMin=[]  SumI3OutMax=[]  SumI4OutMin=[]  SumI4OutMax=[]  SumDOutMin=[]  SumDOutMax=[]  DifferentiatorOutMin=[]  DifferentiatorOutMax=[]  FilterDiffOutCoefMin=[]  FilterDiffOutCoefMax=[]  ReciprocalOutMin=[]  ReciprocalOutMax=[]  SumDenOutMin=[]  SumDenOutMax=[]  SumNumOutMin=[]  SumNumOutMax=[]  DivideOutMin=[]  DivideOutMax=[]  UdiffTsProdOutMin=[]  UdiffTsProdOutMax=[]  NTsProdOutMin=[]  NTsProdOutMax=[]  UintegralTsProdOutMin=[]  UintegralTsProdOutMax=[]  UngainTsProdOutMin=[]  UngainTsProdOutMax=[]  IntegratorContinuousStateAttributes=''  IntegratorStateMustResolveToSignalObject=off  IntegratorRTWStateStorageClass=Auto  FilterContinuousStateAttributes=''  FilterStateMustResolveToSignalObject=off  FilterRTWStateStorageClass=Auto  ParallelPVariant=InternalParameters  IdealPVariant=Disabled  IVariant=InternalParameters  DVariant=InternalParameters  IntegratorVariant=Discrete  SatVariant=Disabled  AWVariant=Passthrough  PCopyVariant=Disabled  TRVariant=Disabled  FdbkBlocksVariant=Forward  IdealPFdbkVariant=Disabled  SatFdbkVariant=Disabled  DerivativeFilterVariant=ForwardEulerFilter  NVariant=InternalParameters  NCopyVariant=Disabled  FilterICVariant=InternalICsFilter  IntegratorICVariant=InternalICs  ExternalResetVariant=Disabled  TRSumVariant=Passthrough  SumFdbkVariant=Disabled  SumVariant=Sum_PID  TsampFilterVariant=InternalTs  TsampNgainVariant=Passthrough  TsampIntegralVariant=Passthrough
  Out1 : Outport  VectorParamsAs1DForOutWhenUnconnected=off
  Out2 : Outport  Port=2  VectorParamsAs1DForOutWhenUnconnected=off
  wires:
  In1/1 -> PID_L/1
  PID_L/1 -> Out1/1
  PID_R/1 -> Out2/1
  In2/1 -> PID_R/1

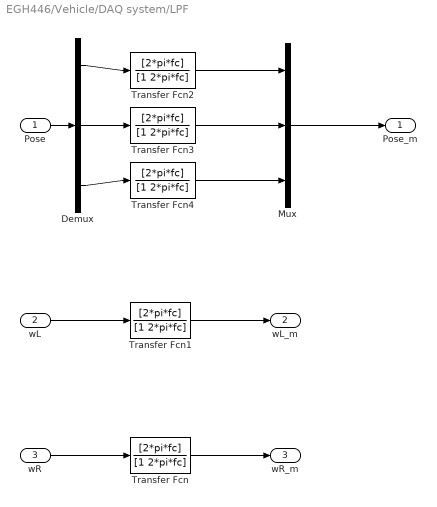
== system EGH446/Vehicle/DAQ system/LPF ==
  Pose : Inport
  wL : Inport  Port=2
  wR : Inport  Port=3
  Demux : Demux  Outputs=3
  Mux : Mux  Inputs=3
  Transfer Fcn{,1..4} (5 alike) : TransferFcn  Numerator=[2*pi*fc]  Denominator=[1 2*pi*fc]
  Pose_m : Outport  VectorParamsAs1DForOutWhenUnconnected=off
  wL_m : Outport  Port=2  VectorParamsAs1DForOutWhenUnconnected=off
  wR_m : Outport  Port=3  VectorParamsAs1DForOutWhenUnconnected=off
  wires:
  Pose/1 -> Demux/1
  Demux/1 -> Transfer Fcn2/1
  Demux/2 -> Transfer Fcn3/1
  Demux/3 -> Transfer Fcn4/1
  Transfer Fcn4/1 -> Mux/3
  Transfer Fcn3/1 -> Mux/2
  Transfer Fcn2/1 -> Mux/1
  Mux/1 -> Pose_m/1
  wL/1 -> Transfer Fcn1/1
  wR/1 -> Transfer Fcn/1
  Transfer Fcn1/1 -> wL_m/1
  Transfer Fcn/1 -> wR_m/1

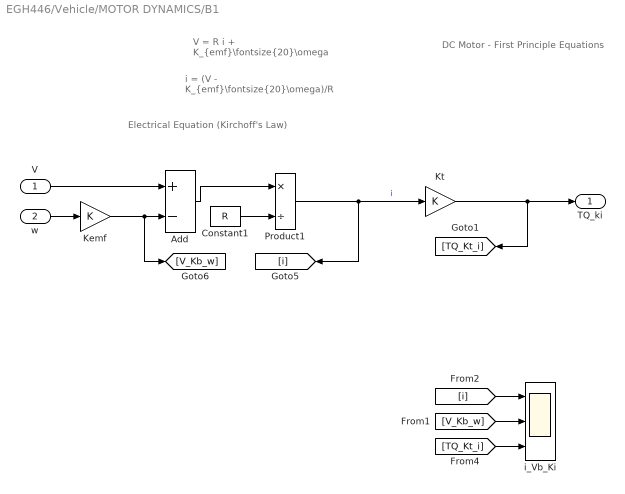
== system EGH446/Vehicle/MOTOR DYNAMICS/B1 ==
  note: Electrical Equation
      | (Kirchoff's Law)
  note: DC Motor - First Principle Equations
  note: V = R i + K_{emf}\fontsize{20}\omega
  note: i = (V - K_{emf}\fontsize{20}\omega)/R
  V : Inport
  w : Inport  Port=2
  Add : Sum  Inputs=+-
  Constant1 : Constant  Value=R
  Kemf : Gain  Gain=K
  Kt : Gain  Gain=K
  Product1 : Product  Inputs=*/
  i_Vb_Ki : Scope  NumInputPorts=3
  TQ_ki : Outport  VectorParamsAs1DForOutWhenUnconnected=off
  wires:
  V/1 -> Add/1
  Product1/1 -> Kt/1, [i]  "i"
  Add/1 -> Product1/1
  Constant1/1 -> Product1/2
  w/1 -> Kemf/1
  Kemf/1 -> [V_Kb_w], Add/2
  Kt/1 -> TQ_ki/1, [TQ_Kt_i]
  [V_Kb_w] -> i_Vb_Ki/2
  [i] -> i_Vb_Ki/1
  [TQ_Kt_i] -> i_Vb_Ki/3

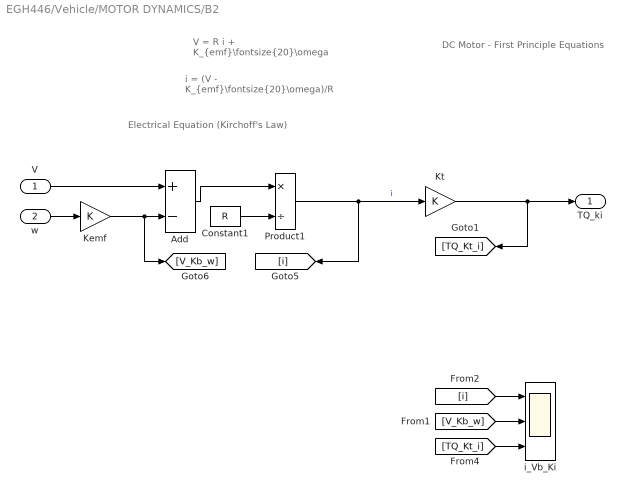
== system EGH446/Vehicle/MOTOR DYNAMICS/B2 ==
  note: Electrical Equation
      | (Kirchoff's Law)
  note: DC Motor - First Principle Equations
  note: V = R i + K_{emf}\fontsize{20}\omega
  note: i = (V - K_{emf}\fontsize{20}\omega)/R
  V : Inport
  w : Inport  Port=2
  Add : Sum  Inputs=+-
  Constant1 : Constant  Value=R
  Kemf : Gain  Gain=K
  Kt : Gain  Gain=K
  Product1 : Product  Inputs=*/
  i_Vb_Ki : Scope  NumInputPorts=3
  TQ_ki : Outport  VectorParamsAs1DForOutWhenUnconnected=off
  wires:
  V/1 -> Add/1
  Product1/1 -> Kt/1, [i]  "i"
  Add/1 -> Product1/1
  Constant1/1 -> Product1/2
  w/1 -> Kemf/1
  Kemf/1 -> [V_Kb_w], Add/2
  Kt/1 -> TQ_ki/1, [TQ_Kt_i]
  [V_Kb_w] -> i_Vb_Ki/2
  [i] -> i_Vb_Ki/1
  [TQ_Kt_i] -> i_Vb_Ki/3

== system EGH446/Vehicle/TQ2VOLTS/B3 ==
  note: V = R.(TQ / K) + K_{emf}\fontsize{20}\omega
  note: TQ = K.i
      | V = R i + K_{emf}\fontsize{20}\omega
  note: DC Motor - First Principle Equations
  note: Assuming SI: K=Kemf
  TQ : Inport
  w : Inport  Port=2
  Add : Sum
  Constant2 : Constant  Value=K
  Kemf : Gain  Gain=K
  Product2 : Product  Inputs=*/
  R : Gain  Gain=R
  V : Outport  VectorParamsAs1DForOutWhenUnconnected=off
  wires:
  R/1 -> Add/1
  Product2/1 -> R/1
  Constant2/1 -> Product2/2
  Kemf/1 -> Add/2
  w/1 -> Kemf/1
  Add/1 -> V/1
  TQ/1 -> Product2/1

== system EGH446/Vehicle/TQ2VOLTS/B4 ==
  note: V = R.(TQ / K) + K_{emf}\fontsize{20}\omega
  note: TQ = K.i
      | V = R i + K_{emf}\fontsize{20}\omega
  note: DC Motor - First Principle Equations
  note: Assuming SI: K=Kemf
  TQ : Inport
  w : Inport  Port=2
  Add : Sum
  Constant2 : Constant  Value=K
  Kemf : Gain  Gain=K
  Product2 : Product  Inputs=*/
  R : Gain  Gain=R
  V : Outport  VectorParamsAs1DForOutWhenUnconnected=off
  wires:
  R/1 -> Add/1
  Product2/1 -> R/1
  Constant2/1 -> Product2/2
  Kemf/1 -> Add/2
  w/1 -> Kemf/1
  Add/1 -> V/1
  TQ/1 -> Product2/1

== matlab function EGH446/Monitor/MATLAB Function ==
  data: vB_C input; vB_A output; theta_dot input; d input
function vB_A = fcn(vB_C, theta_dot, d)

rB_A  = [d,0,0]';
omega = [0,0,theta_dot]';

vB_A = [vB_C(:);0] + cross(omega, rB_A);

== matlab function EGH446/MATLAB Function ==
  data: state input; y output; Xd input; Yd input; vel output; detections input
function [y,vel]  = PID_Control(state, Xd, Yd, detections)

coder.extrinsic('wrapToPi');
persistent previous_error;
persistent integral;
persistent Xo;
persistent Yo;
persistent sign;

Kp =    20;
Ki =    0;
Kd =    30;
Kv =    0.1;
p0 =    1;
Katt =  0;
Krep =  150;

if isempty(integral)
    integral = 0;
    Xo = 100;
    Yo = 100;
    sign = 1;
end


if isempty(previous_error)
    previous_error = 0;
end

%% Calculate Obstacle Position
a = 0;
if ~isempty(detections)
    
    a = atan2(detections(1,2),detections(1,1));
    
    if a>pi
        a = a - 2*pi;
    end
    if a>0 && a<pi
        sign = -1;
    else
        sign = 1;
    end
    d = sqrt(detections(1,1)^2+detections(1,2)^2);
    Xo = state(1)+d*cos(state(3)+a);
    Yo = state(2)+d*sin(state(3)+a);
    
end

%% Calculate Avoidance
d = sqrt((Xo-state(1))^2+(Yo-state(2))^2);
if d < p0 %&& (abs(a)<(3*pi/4))
    Fatt = -Katt*sqrt((Xd-state(1))^2+(Yd-state(2))^2);
    Frep = 0.5* Krep*( ((1/d) - (1/p0))^2)*sign;
    F = Fatt + Frep;
else
    F = 0;
    Xo = inf;
    Yo = inf;    
end


%% Calculate Goal Error
gx = Xd - state(1);
gy = Yd - state(2);
gd = sqrt(gy^2 + gx^2);
error = atan2(gy,gx)-state(3);
if error>pi
    error = error - 2*pi;
end

%% Calculate control
integral = integral +error;
derivative = (error-previous_error);
previous_error = error;
y = (Kp*error)+(Ki*integral)+(Kd*derivative) + F;
vel = max( 0.2+Kv*gd - (F/(sign*10)), 0.2);

== matlab function EGH446/MATLAB Function1 ==
  data: state input; X output; Xd input; Yd input; Y output; detections input; d_error output; stop output
function [X,Y,d_error,stop] = RVWP(state,Xd,Yd, detections)

persistent firstentry
persistent WP_index
coder.extrinsic('wrapToPi');
coder.extrinsic('wrapTo360');
coder.extrinsic('wrapTo2Pi');
coder.extrinsic('RVWP_find');
stop = false;

X = 0;
Y = 0;
d = 0.3;
%%%%%%%
% Upon the first call we need to initialize the variables.
if isempty(firstentry)
    firstentry = 0;
end

if isempty(WP_index)
    WP_index = 0;
end

if firstentry == 0
    WP_index = 2;
    firstentry = 1;
end

%% Check if Finished run
if WP_index > length(Xd)
    stop = true;
    d_error = 0;
else
    %% Begin Choosing Waypoint
    %Extract waypoint list
    Xd(WP_index);
    Yd(WP_index);
    
    %extract vehicle state
    x=state(1);
    y=state(2);
    theta=state(3);
    
    %distance to waypoint
    distance_to_current_waypoint = sqrt((x - Xd(WP_index))^2 + (y - Yd(WP_index))^2);  %WP_index is index for current waypoint
    gx = Xd(WP_index) - state(1);
    gy = Yd(WP_index) - state(2);
    gd = sqrt(gy^2 + gx^2);
    
    d_theta = atan2(gy,gx) - atan2(Yd(WP_index)-Yd(WP_index-1),Xd(WP_index)-Xd(WP_index-1));
    d_error = abs(gd*sin(d_theta));
    
    
    %% Calculate Obstacle Coordinates
    Xo = 100;
    Yo = 100;
    if ~isempty(detections)
        a = atan2(detections(1,2),detections(1,1));
        d = sqrt(detections(1,1)^2+detections(1,2)^2);
        Xo = state(1)+d*cos(state(3)+a);
        Yo = state(2)+d*sin(state(3)+a);
    end
    
    %% Extract Current WP
    X = Xd(WP_index);
    Y = Yd(WP_index);
    
    %% Check and Switch WP if WP is reached, or if WP is within range of Obstacle
    dWP_Ob = sqrt((Xo - Xd(WP_index))^2 + (Yo - Yd(WP_index))^2);
    if distance_to_current_waypoint < 0.15 || dWP_Ob < 0.5
        WP_index = WP_index+1;
    else
        WP_index = WP_index;
    end
    
end
